simulink model "model2"  (R2021a)
settings: Solver=VariableStepAuto  StartTime=0.0  StopTime=10.0  RelTol=1e-3
values from neighbouring files (symbols this model uses):
  A_1 = 20    [skripta.m]
  A_2 = 20    [skripta.m]
  A_c = 250e-4    (= 0.025)    [skripta.m]
  g = 9.81    [skripta.m]
  H_u1 = 4    [skripta.m]
  H_u2 = 4    [skripta.m]
  K_v = 0.5/0.01/60    (= 0.833333333333)    [skripta.m]
settings Model: Creator=Luka  LastModifiedBy=Luka

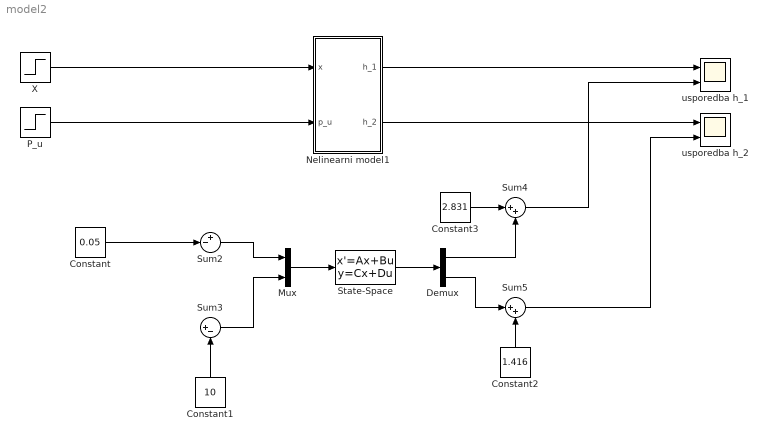
== system model2 ==
  Constant : Constant  Value=0.05
  Constant1 : Constant  Value=10
  Constant2 : Constant  Value=1.416
  Constant3 : Constant  Value=2.831
  Demux : Demux  Outputs=2
  Mux : Mux  Inputs=2
  Nelinearni model1 : Subsystem
  P_u : Step  Time=15000  Before=10  After=10-10*0.4  SampleTime=0
  State-Space : StateSpace  InitialCondition=0
  Sum2 : Sum  Inputs=+-|
  Sum3 : Sum  Inputs=|+-
  Sum4 : Sum  Inputs=|++
  Sum5 : Sum  Inputs=|++
  X : Step  Time=5000  Before=0.05  After=0.05+0.05*0.1  SampleTime=0
  usporedba h_1 : Scope  NumInputPorts=2
  usporedba h_2 : Scope  NumInputPorts=2
  wires:
  P_u/1 -> Nelinearni model1/2(p_u)
  X/1 -> Nelinearni model1/1(x)
  Sum3/1 -> Mux/2
  Sum2/1 -> Mux/1
  Constant2/1 -> Sum5/2
  Constant3/1 -> Sum4/1
  Sum4/1 -> usporedba h_1/2
  Demux/1 -> Sum4/2
  Sum5/1 -> usporedba h_2/2
  Nelinearni model1/2(h_2) -> usporedba h_2/1
  Nelinearni model1/1(h_1) -> usporedba h_1/1
  Constant1/1 -> Sum3/2
  Mux/1 -> State-Space/1
  Demux/2 -> Sum5/1
  Constant/1 -> Sum2/2
  State-Space/1 -> Demux/1

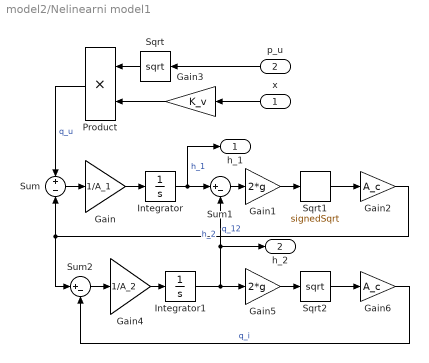
== system model2/Nelinearni model1 ==
  x : Inport
  p_u : Inport  Port=2
  Gain : Gain  Gain=1/A_1
  Gain1 : Gain  Gain=2*g
  Gain2 : Gain  Gain=A_c
  Gain3 : Gain  Gain=K_v
  Gain4 : Gain  Gain=1/A_2
  Gain5 : Gain  Gain=2*g
  Gain6 : Gain  Gain=A_c
  Integrator : Integrator  InitialCondition=2.831  LimitOutput=on  UpperSaturationLimit=H_u1  LowerSaturationLimit=0
  Integrator1 : Integrator  InitialCondition=1.416  LimitOutput=on  UpperSaturationLimit=H_u2  LowerSaturationLimit=0
  Product : Product
  Sqrt : Sqrt  OutputSignalType=real  SaturateOnIntegerOverflow=on
  Sqrt1 : Sqrt  Operator=signedSqrt  OutputSignalType=real  SaturateOnIntegerOverflow=on
  Sqrt2 : Sqrt  OutputSignalType=real  SaturateOnIntegerOverflow=on
  Sum : Sum  Inputs=+-
  Sum1 : Sum  Inputs=|+-
  Sum2 : Sum  Inputs=|+-
  h_1 : Outport
  h_2 : Outport  Port=2
  wires:
  Gain3/1 -> Product/2
  Sqrt/1 -> Product/1
  Product/1 -> Sum/1  "q_u"
  p_u/1 -> Sqrt/1
  x/1 -> Gain3/1
  Gain2/1 -> Sum2/1, Sum/2  "q_12"
  Sum1/1 -> Gain1/1
  Gain1/1 -> Sqrt1/1
  Sqrt1/1 -> Gain2/1
  Gain6/1 -> Sum2/2  "q_i"
  Gain4/1 -> Integrator1/1
  Gain/1 -> Integrator/1
  Gain5/1 -> Sqrt2/1
  Sqrt2/1 -> Gain6/1
  Sum/1 -> Gain/1
  Integrator/1 -> h_1/1, Sum1/1  "h_1"
  Sum2/1 -> Gain4/1
  Integrator1/1 -> h_2/1, Sum1/2, Gain5/1  "h_2"
